simulink model "MBKwithLQR"  (R2018a)
settings: Solver=ode4  StartTime=0.0  StopTime=10  FixedStep=0.01  RelTol=1e-3
values from neighbouring files (symbols this model uses):
  b = 2    [MBK.m]
  k = 5    [MBK.m]
  m = 10    [MBK.m]
settings Model: Creator=Ali  LastModifiedBy=Ali

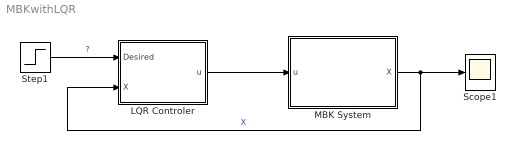
== system MBKwithLQR ==
  LQR Controler : Subsystem
  MBK System : Subsystem
  Scope1 : Scope
  Step1 : Step  After=6  SampleTime=0
  wires:
  MBK System/1(X) -> LQR Controler/2(X), Scope1/1  "X"
  Step1/1 -> LQR Controler/1(Desired)  "?"
  LQR Controler/1(u) -> MBK System/1(u)

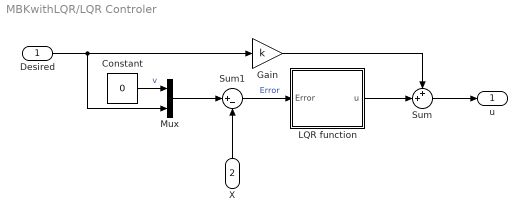
== system MBKwithLQR/LQR Controler ==
  Desired : Inport
  X : Inport  Port=2
  Constant : Constant  Value=0
  Gain : Gain  Gain=k
  LQR function : MATLAB Function  TreatAsAtomicUnit=on
  Mux : Mux  Inputs=2
  Sum : Sum  Inputs=++|
  Sum1 : Sum  Inputs=|+-
  u : Outport
  wires:
  X/1 -> Sum1/2
  Mux/1 -> Sum1/1
  LQR function/1(u) -> Sum/2
  Constant/1 -> Mux/1  "v"
  Sum/1 -> u/1
  Sum1/1 -> LQR function/1(Error)  "Error"
  Gain/1 -> Sum/1
  Desired/1 -> Gain/1, Mux/2

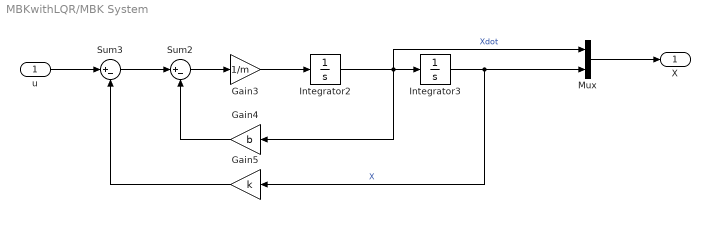
== system MBKwithLQR/MBK System ==
  u : Inport
  Gain3 : Gain  Gain=1/m
  Gain4 : Gain  Gain=b
  Gain5 : Gain  Gain=k
  Integrator2 : Integrator
  Integrator3 : Integrator  InitialCondition=3
  Mux : Mux  Inputs=2
  Sum2 : Sum  Inputs=|+-
  Sum3 : Sum  Inputs=|+-
  X : Outport
  wires:
  u/1 -> Sum3/1
  Gain4/1 -> Sum2/2
  Gain3/1 -> Integrator2/1
  Integrator3/1 -> Mux/2, Gain5/1  "X"
  Gain5/1 -> Sum3/2
  Sum2/1 -> Gain3/1
  Integrator2/1 -> Mux/1, Gain4/1, Integrator3/1  "Xdot"
  Sum3/1 -> Sum2/1
  Mux/1 -> X/1

== matlab function MBKwithLQR/LQR Controler/LQR function ==
  settings: updateMethod=DISCRETE
  data: u output; Error input
function u = LQR(Error)
m = 10;
b = 2;
k = 5;
A = [0    1;
   -k/m -b/m];
B = [0; 1/m];
H = [2 0;...
     0 0];
Q = [2000 0;...
     0 10] ;
R = 0.1;
Ts = 0.001 ;
Tf = 2 ; 
t = 0:Ts:Tf ;
N = numel(t) ;
P = zeros(2 , 2 , N);
P(:,:,N) = H ; 
persistent Forloop;
persistent pp;
if isempty(Forloop)
    Forloop = 1;
    for k = N-1:-1:2
        P(:,:,k-1) = P(: , : , k) + Ts*(Q -P(: , : , k)*B*R^(-1)*B'*P(: , : , k)+P(: , : , k)*A+A'*P(: , : , k)) ;
    end
    pp = P(:, :, 1);
end
Temp = zeros(2, 1);
Temp(1) = Error(2, 1);
Temp(2) = Error(1, 1);
K = -R^(-1)*B'*pp;
u = -K*Temp;
